simulink model "ELIPSE_Data_ETR07"  (R2017b)
settings: Solver=FixedStepAuto  StartTime=0.0  StopTime=10.0  RelTol=1e-3
settings Model: Creator=cspt  LastModifiedBy=cspt
settings RTWCC: SystemTargetFile=irt.tlc  TemplateMakefile=irt_default_tmf  Description=INTECRIO Real-Time Target
settings STFCustomTargetCC: TargetLangStandard=C99 (ISO)  UtilityFuncGeneration=Shared location  SystemTargetFile=irt.tlc
settings GRTTargetCC: UtilityFuncGeneration=Shared location  ParMdlRefBuildCompliant=off  CompOptLevelCompliant=off  ConcurrentExecutionCompliant=off  CombineOutputUpdateFcns=off  MatFileLogging=off  CPPClassGenCompliant=off  GRTInterface=on  UseToolchainInfoCompliant=off  GenerateASAP2=on

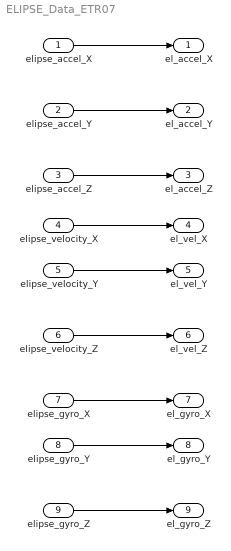
== system ELIPSE_Data_ETR07 ==
  elipse_accel_X : Inport
  elipse_accel_Y : Inport  Port=2
  elipse_accel_Z : Inport  Port=3
  elipse_velocity_X : Inport  Port=4
  elipse_velocity_Y : Inport  Port=5
  elipse_velocity_Z : Inport  Port=6
  elipse_gyro_X : Inport  Port=7
  elipse_gyro_Y : Inport  Port=8
  elipse_gyro_Z : Inport  Port=9
  el_accel_X : Outport
  el_accel_Y : Outport  Port=2
  el_accel_Z : Outport  Port=3
  el_vel_X : Outport  Port=4
  el_vel_Y : Outport  Port=5
  el_vel_Z : Outport  Port=6
  el_gyro_X : Outport  Port=7
  el_gyro_Y : Outport  Port=8
  el_gyro_Z : Outport  Port=9
  wires:
  elipse_velocity_Z/1 -> el_vel_Z/1
  elipse_velocity_Y/1 -> el_vel_Y/1
  elipse_velocity_X/1 -> el_vel_X/1
  elipse_accel_Z/1 -> el_accel_Z/1
  elipse_accel_Y/1 -> el_accel_Y/1
  elipse_accel_X/1 -> el_accel_X/1
  elipse_gyro_X/1 -> el_gyro_X/1
  elipse_gyro_Y/1 -> el_gyro_Y/1
  elipse_gyro_Z/1 -> el_gyro_Z/1
